simulink model "SolarTracker"  (R2019b)
settings: Solver=VariableStepAuto  StartTime=0.0  StopTime=10.0  RelTol=1e-3
model workspace (MAT data in the model file):
  J = 8.6
  Kd = 5
  Kf = 0.07
  Kg = 2000
  Kt = 0.07
  L = 1e-05
  R = 10
libraries: simulink x1
settings Model: Creator=haider  LastModifiedBy=haider

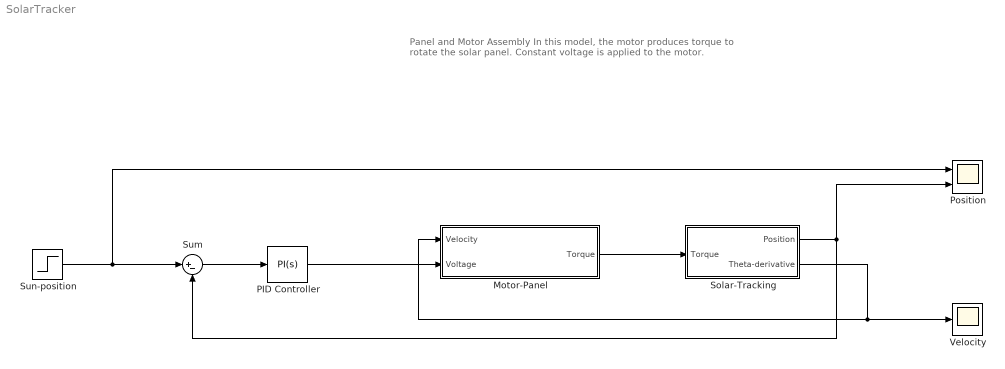
== system SolarTracker ==
  note: Panel and Motor Assembly
      |
      | In this model, the motor produces torque to rotate the solar panel. Constant voltage is applied to the motor.
  Motor-Panel : Subsystem
  PID Controller : simulink/Continuous/PID Controller  Controller=PI  Form=Parallel  TimeDomain=Continuous-time  SampleTime=-1  IntegratorMethod=Forward Euler  FilterMethod=Forward Euler  ControllerParametersSource=internal  P=240  I=180  D=0  UseFilter=on  N=100  TunerSelectOption=Transfer Function Based (PID Tuner App)  InitialConditionSource=internal  InitialConditionForIntegrator=0  InitialConditionForFilter=0  DifferentiatorICPrevScaledInput=0  ExternalReset=none  TrackingMode=off  Kt=1  LimitOutput=off  UpperSaturationLimit=inf  LowerSaturationLimit=-inf  LinearizeAsGain=on  AntiWindupMode=none  Kb=1  POutMin=[]  POutMax=[]  IOutMin=[]  IOutMax=[]  DOutMin=[]  DOutMax=[]  NOutMin=[]  NOutMax=[]  SumOutMin=[]  SumOutMax=[]  SaturationOutMin=[]  SaturationOutMax=[]  PParamMin=[]  PParamMax=[]  IParamMin=[]  IParamMax=[]  DParamMin=[]  DParamMax=[]  NParamMin=[]  NParamMax=[]  KbParamMin=[]  KbParamMax=[]  KtParamMin=[]  KtParamMax=[]  KbOutMin=[]  KbOutMax=[]  KtOutMin=[]  KtOutMax=[]  IntegratorOutMin=[]  IntegratorOutMax=[]  FilterOutMin=[]  FilterOutMax=[]  SumI1OutMin=[]  SumI1OutMax=[]  SumI2OutMin=[]  SumI2OutMax=[]  SumI3OutMin=[]  SumI3OutMax=[]  SumI4OutMin=[]  SumI4OutMax=[]  SumDOutMin=[]  SumDOutMax=[]  DifferentiatorOutMin=[]  DifferentiatorOutMax=[]  FilterDiffOutCoefMin=[]  FilterDiffOutCoefMax=[]  ReciprocalOutMin=[]  ReciprocalOutMax=[]  SumDenOutMin=[]  SumDenOutMax=[]  SumNumOutMin=[]  SumNumOutMax=[]  DivideOutMin=[]  DivideOutMax=[]  IntegratorContinuousStateAttributes=''  IntegratorStateMustResolveToSignalObject=off  IntegratorRTWStateStorageClass=Auto  FilterContinuousStateAttributes=''  FilterStateMustResolveToSignalObject=off  FilterRTWStateStorageClass=Auto  ParallelPVariant=InternalParameters  IdealPVariant=Disabled  IVariant=InternalParameters  DVariant=Disabled  IntegratorVariant=Continuous  SatVariant=Disabled  AWVariant=Passthrough  PCopyVariant=Disabled  TRVariant=Disabled  FdbkBlocksVariant=Forward  IdealPFdbkVariant=Disabled  SatFdbkVariant=Disabled  DerivativeFilterVariant=Disabled  NVariant=Disabled  NCopyVariant=Disabled_SignalSpec  FilterICVariant=Disabled  IntegratorICVariant=InternalICs  ExternalResetVariant=Disabled  TRSumVariant=Passthrough  SumFdbkVariant=Disabled  SumVariant=Sum_PI
  "Position " : Scope  NumInputPorts=2
  Solar-Tracking : Subsystem
  Sum : Sum  Inputs=|+-
  Sun-position : Step  SampleTime=0
  "Velocity " : Scope
  wires:
  Solar-Tracking/1(Position) -> Sum/2, "Position "/2
  Solar-Tracking/2(Theta-derivative) -> "Velocity "/1, Motor-Panel/1(Velocity)
  PID Controller/1 -> Motor-Panel/2(Voltage)
  Motor-Panel/1(Torque) -> Solar-Tracking/1("Torque ")
  Sum/1 -> PID Controller/1
  Sun-position/1 -> "Position "/1, Sum/1

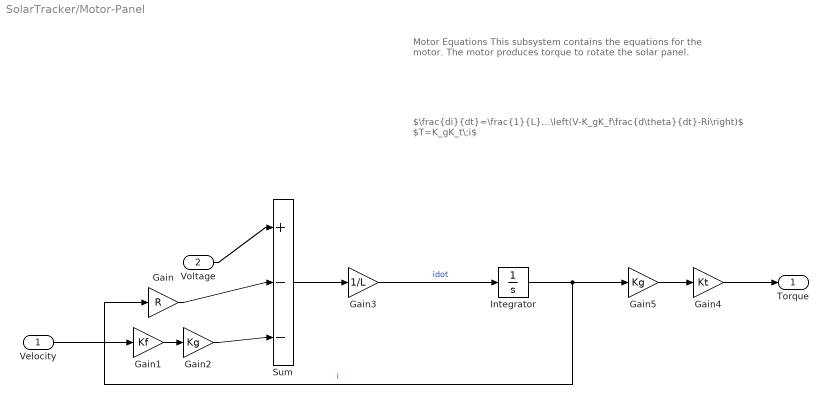
== system SolarTracker/Motor-Panel ==
  note: $\frac{di}{dt}=\frac{1}{L}\left(V-K_gK_f\frac{d\theta}{dt}-Ri\right)$
      | $T=K_gK_t\;i$
  note: Motor Equations
      |
      | This subsystem contains the equations for the motor. The motor produces torque to rotate the solar panel.
  Velocity : Inport
  Voltage : Inport  Port=2
  Gain : Gain  Gain=R
  Gain1 : Gain  Gain=Kf
  Gain2 : Gain  Gain=Kg
  Gain3 : Gain  Gain=1/L
  Gain4 : Gain  Gain=Kt
  Gain5 : Gain  Gain=Kg
  Integrator : Integrator
  Sum : Sum  Inputs=|+--
  Torque : Outport
  wires:
  Integrator/1 -> Gain5/1, Gain/1  "i"
  Gain2/1 -> Sum/3
  Gain/1 -> Sum/2
  Velocity/1 -> Gain1/1
  Gain1/1 -> Gain2/1
  Voltage/1 -> Sum/1
  Sum/1 -> Gain3/1
  Gain3/1 -> Integrator/1  "idot"
  Gain5/1 -> Gain4/1
  Gain4/1 -> Torque/1

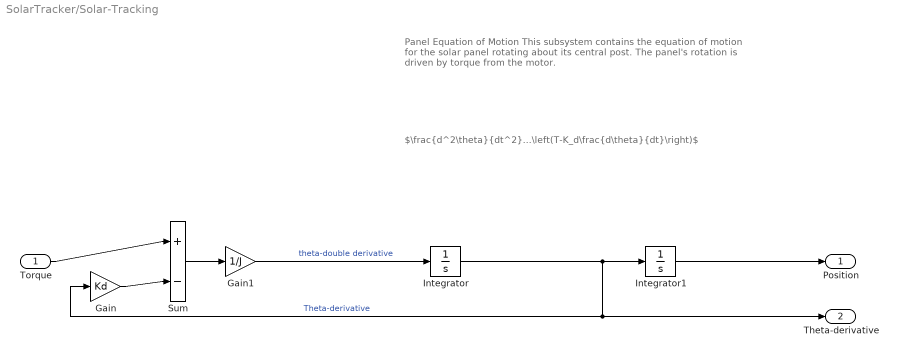
== system SolarTracker/Solar-Tracking ==
  note: Panel Equation of Motion
      |
      | This subsystem contains the equation of motion for the solar panel rotating about its central post. The panel's rotation is driven by torque from the motor.
  note: $\frac{d^2\theta}{dt^2}=\frac{1}{J}\left(T-K_d\frac{d\theta}{dt}\right)$
  "Torque " : Inport
  Gain : Gain  Gain=Kd
  Gain1 : Gain  Gain=1/J
  Integrator : Integrator
  Integrator1 : Integrator
  Sum : Sum  Inputs=|+-
  Position : Outport
  Theta-derivative : Outport  Port=2
  wires:
  Integrator/1 -> Gain/1, Theta-derivative/1, Integrator1/1  "Theta-derivative"
  Sum/1 -> Gain1/1
  Gain/1 -> Sum/2
  "Torque "/1 -> Sum/1
  Integrator1/1 -> Position/1
  Gain1/1 -> Integrator/1  "theta-double derivative"
